simulink model "rc_coder"  (R2019b)
settings: Solver=FixedStepDiscrete  StartTime=0.0  StopTime=Inf  FixedStep=0.025  RelTol=1e-3  EnableMultiTasking=on
PreLoadFcn:
  | mdlname = bdroot;
  | oldFolder = cd(fileparts(which(mdlname)));
  | % cd ..\
  | 
  | load('./bus_type/bus_type.mat');
model workspace (MAT data in the model file):
  ADCDRES : Simulink.Parameter (value not decoded)
  ADCSRES : Simulink.Parameter (value not decoded)
  CLK : Simulink.Parameter (value not decoded)
  EncoderScaler : Simulink.Parameter (value not decoded)
  GearBoxScaler : Simulink.Parameter (value not decoded)
  Kd_T : Simulink.Parameter (value not decoded)
  Kd_theta : Simulink.Parameter (value not decoded)
  Ki_T : Simulink.Parameter (value not decoded)
  Ki_theta : Simulink.Parameter (value not decoded)
  Kp_T : Simulink.Parameter (value not decoded)
  Kp_theta : Simulink.Parameter (value not decoded)
  LowerTempLimitHigh : Simulink.Parameter (value not decoded)
  LowerTempLimitLow : Simulink.Parameter (value not decoded)
  MinMeasurableSpd : Simulink.Parameter (value not decoded)
  ModePWM : Simulink.Parameter (value not decoded)
  ModePosition : Simulink.Parameter (value not decoded)
  ModePrecool : Simulink.Parameter (value not decoded)
  ModeTemp : Simulink.Parameter (value not decoded)
  PWMFreq : Simulink.Parameter (value not decoded)
  QuadratureEncScaler : Simulink.Parameter (value not decoded)
  S1DelaySeconds : Simulink.Parameter (value not decoded)
  S2DelaySeconds : Simulink.Parameter (value not decoded)
  S3DelaySeconds : Simulink.Parameter (value not decoded)
  S4DelaySeconds : Simulink.Parameter (value not decoded)
  SamplingR : Simulink.Parameter (value not decoded)
  StepSize : Simulink.Parameter (value not decoded)
  TErrBand : Simulink.Parameter (value not decoded)
  ThetaErrBand : Simulink.Parameter (value not decoded)
  VADCREF : Simulink.Parameter (value not decoded)
symbols that are objects in the model workspace (value not decoded): ADCDRES, CLK, EncoderScaler, GearBoxScaler, Kd_T, Kd_theta, Ki_T, Ki_theta, Kp_T, Kp_theta, LowerTempLimitHigh, LowerTempLimitLow, MinMeasurableSpd, ModePosition, ModePrecool, ModePWM, ModeTemp, PWMFreq, QuadratureEncScaler, S1DelaySeconds, S2DelaySeconds, S3DelaySeconds, S4DelaySeconds, StepSize, TErrBand, ThetaErrBand
undefined symbols (not defined in the file or in its folder): DiscIntNeverNeededParam, Down, GPTRIP1SEL, GPTRIP2SEL, TZ1, TZ2, Up
libraries: simulink x21, c2802xlib x12, c2837xDlib x10, c280xlib x9, dspstat3 x8, dspfdesign x7, commutil2 x3, c2000lib x2
(part 4 of 4)

== system rc_coder/Sensing/Incremental Encoder/CalcSpd1/zero_spd_check/Subsystem ==
  poscnt : Inport
  Detect Change : simulink/Logic and Bit Operations/Detect Change  vinit=0  OutDataTypeStr=boolean
  If : If  IfExpression=u1 == 1
  If Action Subsystem : Subsystem  TreatAsAtomicUnit=on
  If Action Subsystem1 : Subsystem  TreatAsAtomicUnit=on
  Merge : Merge
  Saturation : Saturate  UpperLimit=60 / (MinMeasurableSpd * EncoderScaler) / StepSize +100  LowerLimit=0
  Unit Delay1 : UnitDelay  SampleTime=-1  HasFrameUpgradeWarning=on
  no_measurement_cnt : Outport
  wires:
  Saturation/1 -> no_measurement_cnt/1
  poscnt/1 -> Detect Change/1
  If/1 -> If Action Subsystem/Action
  If/2 -> If Action Subsystem1/Action
  If Action Subsystem1/1(Out1) -> Merge/2
  If Action Subsystem/1(Out1) -> Merge/1
  Unit Delay1/1 -> If Action Subsystem1/1(In1)
  Detect Change/1 -> If/1
  Merge/1 -> Saturation/1, Unit Delay1/1

== system rc_coder/Sensing/Incremental Encoder/CalcSpd1/zero_spd_check/Subsystem1 ==
  spd_last_measurement : Inport
  Constant1 : Constant  Value=60 / (MinMeasurableSpd * EncoderScaler)
  Constant5 : Constant  Value=2 * pi / EncoderScaler
  Divide2 : Product  Inputs=*/
  Gain : Gain  Gain=1 / StepSize
  MinMax : MinMax  Inputs=2
  cnts_to_wait : Outport
  wires:
  Constant1/1 -> MinMax/2
  MinMax/1 -> Gain/1
  Gain/1 -> cnts_to_wait/1
  Divide2/1 -> MinMax/1
  spd_last_measurement/1 -> Divide2/2
  Constant5/1 -> Divide2/1

== system rc_coder/Sensing/Incremental Encoder/CalcSpd/zero_spd_check/Subsystem/If Action Subsystem ==
  Action Port : ActionPort  ActionPortLabel=if(u1 == 1)
  Constant : Constant  Value=0
  Out1 : Outport
  wires:
  Constant/1 -> Out1/1

== system rc_coder/Sensing/Incremental Encoder/CalcSpd/zero_spd_check/Subsystem/If Action Subsystem1 ==
  In1 : Inport
  Action Port : ActionPort  ActionPortLabel=else
  Increment Real World : simulink/Additional Math & Discrete/Additional Math: Increment - Decrement/Increment Real World
      settings: SourceProductName=Simulink  SourceProductBaseCode=SL
  Out1 : Outport
  wires:
  In1/1 -> Increment Real World/1
  Increment Real World/1 -> Out1/1

== system rc_coder/Sensing/Incremental Encoder/CalcSpd1/zero_spd_check/Subsystem/If Action Subsystem ==
  Action Port : ActionPort  ActionPortLabel=if(u1 == 1)
  Constant : Constant  Value=0
  Out1 : Outport
  wires:
  Constant/1 -> Out1/1

== system rc_coder/Sensing/Incremental Encoder/CalcSpd1/zero_spd_check/Subsystem/If Action Subsystem1 ==
  In1 : Inport
  Action Port : ActionPort  ActionPortLabel=else
  Increment Real World : simulink/Additional Math & Discrete/Additional Math: Increment - Decrement/Increment Real World
      settings: SourceProductName=Simulink  SourceProductBaseCode=SL
  Out1 : Outport
  wires:
  Increment Real World/1 -> Out1/1
  In1/1 -> Increment Real World/1

== stateflow chart rc_coder/CiA 402 ==
  state OPERATION_ENABLE
    entry:
    OutBus.EnableActr1 = 1;
    OutBus.EnableActr2 = 1;
    status = 52;
    exit:
    ;
    state POSITION_MODE
      entry:
      OutBus.Cmd1 = command(2);
      OutBus.Cmd2 = command(3);
      status = ModePosition;
    state IDLE_MODE
      entry:
      OutBus.Cmd1 = command(2);
      OutBus.Cmd2 = command(3);
      OutBus.Cmd3 = command(4);
      OutBus.Cmd4 = command(5);
      status = 52;
    state SPEED_MODE [commented out]
      entry:
      OutBus.SpeedCommand1 = command(2);
      OutBus.SpeedCommand2 = command(3);
    state TEMP_MODE
      entry:
      OutBus.Cmd1 = command(2);
      OutBus.Cmd2 = command(3);
      OutBus.Cmd3 = command(4);
      OutBus.Cmd4 = command(5);
      status = ModeTemp;
    state PWM_MODE
      entry:
      OutBus.Cmd1 = command(2);
      OutBus.Cmd2 = command(3);
      OutBus.Cmd3 = command(4);
      OutBus.Cmd4 = command(5);
      status = ModePWM;
    state PRECOOL_MODE
      entry:
      OutBus.Cmd1 = command(2);
      OutBus.Cmd2 = command(3);
      OutBus.Cmd3 = command(4);
      OutBus.Cmd4 = command(5);
      status = ModePrecool;
    POSITION_MODE -> POSITION_MODE [order 2] : [command(1) == 100]
    (default) -> IDLE_MODE
    IDLE_MODE -> POSITION_MODE [order 1] : [command(1) == 14]
    POSITION_MODE -> IDLE_MODE [order 1] : [command(1) == 15]
    SPEED_MODE -> SPEED_MODE [commented out] : [command(1) == 160]
    IDLE_MODE -> SPEED_MODE [commented out] : [command(1) == 16]
    SPEED_MODE -> IDLE_MODE [commented out] : [command(1) == 17]
    TEMP_MODE -> TEMP_MODE [order 2] : [command(1) == 100]
    IDLE_MODE -> TEMP_MODE [order 4] : [command(1) == 18]
    TEMP_MODE -> IDLE_MODE [order 1] : [command(1) == 19]
    PWM_MODE -> PWM_MODE [order 2] : [command(1) == 100]
    IDLE_MODE -> PWM_MODE [order 3] : [command(1) == 20]
    PWM_MODE -> IDLE_MODE [order 1] : [command(1) == 21]
    PRECOOL_MODE -> PRECOOL_MODE [order 2] : [command(1) == 100]
    IDLE_MODE -> PRECOOL_MODE [order 2] : [command(1) == 22]
    PRECOOL_MODE -> IDLE_MODE [order 1] : [command(1) == 23]
  state READY_TO_SWITCH_ON
    entry:
    OutBus.EnableActr1 = 0;
    OutBus.EnableActr2 = 0;
    status = 50;
    exit:
    ;
  state SWITCHED_ON
    entry:
    OutBus.EnableActr1 = 0;
    OutBus.EnableActr2 = 0;
    status = 51;
    exit:
    ;
  OPERATION_ENABLE -> READY_TO_SWITCH_ON [order 2] : [command(1) == 0]
  SWITCHED_ON -> READY_TO_SWITCH_ON [order 3] : [command(1) == 0]
  (default) -> READY_TO_SWITCH_ON
  SWITCHED_ON -> OPERATION_ENABLE [order 2] : [command(1) == 12]
  READY_TO_SWITCH_ON -> SWITCHED_ON : [command(1) == 10]
  SWITCHED_ON -> READY_TO_SWITCH_ON [order 1] : [command(1) == 11]
  OPERATION_ENABLE -> SWITCHED_ON [order 1] : [command(1) == 13]
  data: status output single; command input; OutBus output Bus: StateMachinOutBus; ModePosition parameter; ModePrecool parameter; ModePWM parameter; ModeTemp parameter
